simulink model "mysvm"  (R2017b)
settings: Solver=ode45  StartTime=0.0  StopTime=0.02  RelTol=1e-3  EnableMultiTasking=on
values from neighbouring files (symbols this model uses):
  N = svminput(5) - 1    [MLSVM_m_HD.m]    (also in PlotSpaceVector.m = block.DialogPrm(1).Data - 1)
undefined symbols (not defined in the file or in its folder): m
libraries: powerlib x9, powerlib_meascontrol x5, simulink x1
settings Model: Creator=吴鸿达  LastModifiedBy=AdamWu
settings DataIOCC: LimitDataPoints=on  SaveFormat=Array  ReturnWorkspaceOutputs=on
settings OptimizationCC: LifeSpan=inf
settings DebuggingCC: SolverPrmCheckMsg=warning  SFUnexpectedBacktrackingDiag=warning  SFNoUnconditionalDefaultTransitionDiag=warning  SFExecutionAtInitializationDiag=none
settings HardwareCC: ProdBitPerPointer=32  ProdBitPerSizeT=32  ProdBitPerPtrDiffT=32  ProdLargestAtomicFloat=None  ProdIntDivRoundTo=Undefined  ProdEndianess=Unspecified  ProdWordSize=32  ProdHWDeviceType=32-bit Generic
settings ModelReferenceCC: PropagateSignalLabelsOutOfModel=off
settings CodeAppCC: StateflowObjectComments=on
settings GRTTargetCC: TargetLangStandard=C89/C90 (ANSI)  GeneratePreprocessorConditionals=Disable all
settings ConfigComp: CovMetricSettings=dw  CovHtmlReporting=on  CovSaveCumulativeToWorkspaceVar=on  CovSaveSingleToWorkspaceVar=on  CovExternalEMLEnable=off  CovSFcnEnable=off
settings SimscapeCC: SimscapeNormalizeSystem=off

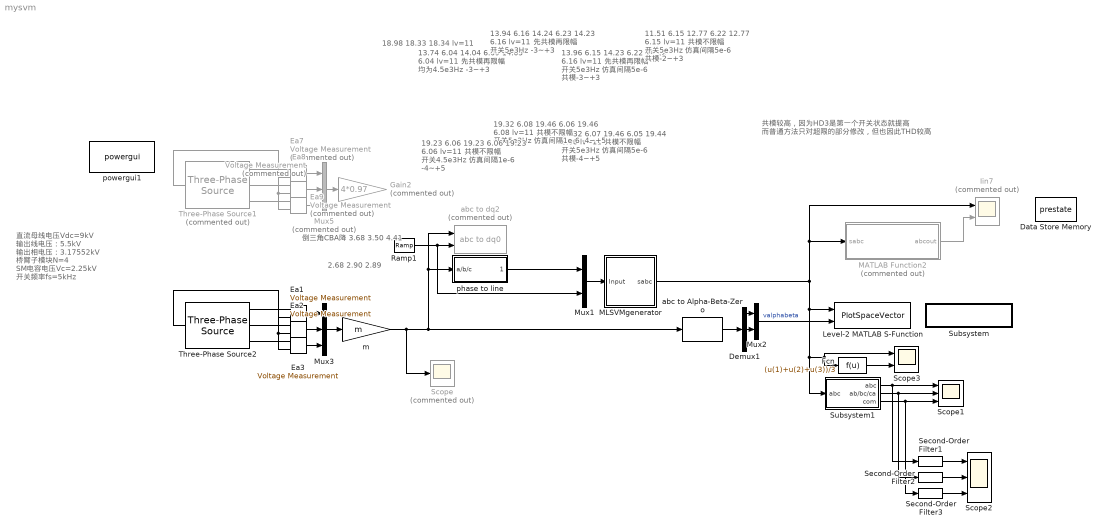
== system mysvm ==
  note: 18.98
      | 18.33
      | 18.34
      | lv=11
  note: 2.68 2.90 2.89
  note: 直流母线电压Vdc=9kV
      |
      | 输出线电压：5.5kV
      | 输出相电压：3.17552kV
      | 桥臂子模块N=4
      | SM电容电压Vc=2.25kV
      | 开关频率fs=5kHz
  note: 倒三角CBA降 3.68 3.50 4.41
  note: 13.74	6.04
      | 14.04	6.09
      | 14.05	6.04
      | lv=11
      | 先共模再限幅
      | 均为4.5e3Hz
      | -3~+3
  note: 13.94	6.16
      | 14.24	6.23
      | 14.23	6.16
      | lv=11
      | 先共模再限幅
      | 开关5e3Hz
      | -3~+3
  note: 13.96	6.15
      | 14.23	6.22
      | 14.22	6.16
      | lv=11
      | 先共模再限幅
      | 开关5e3Hz
      | 仿真间隔5e-6
      | 共模-3~+3
  note: 19.32	6.07
      | 19.46	6.05
      | 19.44	6.08
      | lv=11
      | 共模不限幅
      | 开关5e3Hz
      | 仿真间隔5e-6
      | 共模-4~+5
  note: 19.32	6.08
      | 19.46	6.06
      | 19.46	6.08
      | lv=11
      | 共模不限幅
      | 开关5e3Hz
      | 仿真间隔1e-6
      | -4~+5
  note: 19.23	6.06
      | 19.23	6.06
      | 19.23	6.06
      | lv=11
      | 共模不限幅
      | 开关4.5e3Hz
      | 仿真间隔1e-6
      | -4~+5
  note: 11.51	6.15
      | 12.77	6.22
      | 12.77	6.15
      | lv=11
      | 共模不限幅
      | 开关5e3Hz
      | 仿真间隔5e-6
      | 共模-2~+3
  note: 共模较高，因为HD3是第一个开关状态就提高
      | 而普通方法只对超限的部分修改，但也因此THD较高
  Data Store Memory : DataStoreMemory  DataStoreName=prestate  ReadBeforeWriteMsg=warning  WriteAfterWriteMsg=warning  WriteAfterReadMsg=warning  InitialValue=[0 0 0 0 0 0 0 1 0]  ShowAdditionalParam=off  OutDataTypeStr=double
  Demux1 : Demux  Outputs=3
  Ea1 : powerlib/Measurements/Voltage Measurement  PhasorSimulation=off  OutputType=Complex  PSBequivalent=0
  Ea2 : powerlib/Measurements/Voltage Measurement  PhasorSimulation=off  OutputType=Complex  PSBequivalent=0
  Ea3 : powerlib/Measurements/Voltage Measurement  PhasorSimulation=off  OutputType=Complex  PSBequivalent=0
  Ea7 : powerlib/Measurements/Voltage Measurement  Commented=on  PhasorSimulation=off  OutputType=Complex  PSBequivalent=0
  Ea8 : powerlib/Measurements/Voltage Measurement  Commented=on  PhasorSimulation=off  OutputType=Complex  PSBequivalent=0
  Ea9 : powerlib/Measurements/Voltage Measurement  Commented=on  PhasorSimulation=off  OutputType=Complex  PSBequivalent=0
  Fcn : Fcn  Expr=(u(1)+u(2)+u(3))/3
  Gain2 : Gain  Commented=on  Gain=4*0.97
  Iin7 : Scope  Commented=on  NumInputPorts=2
  Level-2 MATLAB S-Function : M-S-Function  FunctionName=PlotSpaceVector  Parameters=level, vdc, rate, normalized, plot, hexagon, sw, disabled  mask{disabled=off, level=N, rate=100, vdc=2/50, normalized=on, plot=1, hexagon=off, sw=off}
      mask prompts: disabled "Disable Plot"; level "Voltage Level"; rate "Plot Rate"; vdc "DC Link Voltage"; plot "Plot Number"; sw "Show Switching"
  MATLAB Function2 : MATLAB Function  Commented=on  TreatAsAtomicUnit=on
  MLSVMgenerator : Subsystem  mask{level=N, fs=1.5e3, vc=2.25e3, normalized=on, method=H-D3 Axis, dqorline=Line Voltages}
      mask prompts: level "Voltage Level"; fs "Switching Frequency"; vc "Capacitor Voltage"; method "Simplify Algorithm"; dqorline "Input Voltage Type"
      mask TypeOptions method: H-D Axis | g-h Axis | ab-bc-ca Axis | H-D3 Axis | D-Y (v2016) Axis | Rotated H-D Axis (Zero Common Voltage)
      mask TypeOptions dqorline: dq0 Voltages | Line Voltages | Phase Voltages
      mask DialogControl dqorline Tooltip: dq0 voltages means vd vq v0; line voltages means vab vbc vca
  Mux1 : Mux  Inputs=2
  Mux2 : Mux  Inputs=2
  Mux3 : Mux  Inputs=3
  Mux5 : Mux  Commented=on  Inputs=3
  Ramp1 : simulink/Sources/Ramp  slope=2*pi*50  start=0  X0=0
  Scope : Scope  Commented=on
  Scope1 : Scope  NumInputPorts=3
  Scope2 : Scope  NumInputPorts=3
  Scope3 : Scope  NumInputPorts=2
  Second-Order Filter1 : powerlib_meascontrol/Filters/Second-Order Filter  FilterType=Lowpass  Fo=1000  Zeta=0.707  Ts=0  Initialize=on  Vac_Init="[0,  0,  50]"  Vdc_Init=0  PlotResponse=off  FreqRange=[0, 2000, 1]
      settings: SourceProductName=Simscape Power Systems  SourceProductBaseCode=PS
  Second-Order Filter2 : powerlib_meascontrol/Filters/Second-Order Filter  FilterType=Lowpass  Fo=1000  Zeta=0.707  Ts=0  Initialize=on  Vac_Init="[0,  0,  50]"  Vdc_Init=0.5  PlotResponse=off  FreqRange=[0, 2000, 1]
      settings: SourceProductName=Simscape Power Systems  SourceProductBaseCode=PS
  Second-Order Filter3 : powerlib_meascontrol/Filters/Second-Order Filter  FilterType=Lowpass  Fo=1000  Zeta=0.707  Ts=0  Initialize=on  Vac_Init="[0,  0,  50]"  Vdc_Init=0.5  PlotResponse=off  FreqRange=[0, 2000, 1]
      settings: SourceProductName=Simscape Power Systems  SourceProductBaseCode=PS
  Subsystem : Subsystem  mask{filename=SVPWM_sFunction.m}
      settings: AttributesFormatString=\n  OpenFcn=open('F:\研究生\matlab\PlotSpaceVector.m')
      mask Display:
      | patch([0 1 1 0], [0 0 1 1],[0.2 0.6 0.9])
      | disp('plotspacevector.m')
  Subsystem1 : Subsystem  mask{N=N, normal=off}
      mask prompts: N "Voltage Level"; normal "Normalized"
  Three-Phase Source1 : powerlib/Electrical Sources/Three-Phase Source  Commented=on  InternalConnection=Yn  VoltagePhases=off  Voltage=1.59099e3  PhaseAngle=0  Voltage_phases=[25e3 25e3 25e3]/sqrt(3)  PhaseAngles_phases=[0 -120 +120]  Frequency=50  NonIdealSource=off  SpecifyImpedance=off  Resistance=0.8929  Inductance=1e-3  ShortCircuitLevel=100e6  BaseVoltage=25e3  XRratio=7  BusType=swing  Pref=10e3  Qref=0  Prefabc=[10e3, 10e3, 10e3]  Qrefabc=[0, 0, 0]  Qmin=-inf  Qmax=inf
  Three-Phase Source2 : powerlib/Electrical Sources/Three-Phase Source  InternalConnection=Yn  VoltagePhases=off  Voltage=sqrt(2)  PhaseAngle=0  Voltage_phases=[25e3 25e3 25e3]/sqrt(3)  PhaseAngles_phases=[0 -120 +120]  Frequency=50  NonIdealSource=off  SpecifyImpedance=off  Resistance=0.8929  Inductance=1e-3  ShortCircuitLevel=100e6  BaseVoltage=25e3  XRratio=7  BusType=swing  Pref=10e3  Qref=0  Prefabc=[10e3, 10e3, 10e3]  Qrefabc=[0, 0, 0]  Qmin=-inf  Qmax=inf
  abc to Alpha-Beta-Zero : powerlib_meascontrol/Transformations/abc to Alpha-Beta-Zero
      settings: SourceProductName=Simscape Power Systems
  abc to dq2 : powerlib_meascontrol/Transformations/abc to dq0  Commented=on  Alignment=90 degrees behind phase A axis
  m : Gain  Gain=m
  phase to line : Subsystem
  powergui1 : powerlib/powergui  Priority=1  SimulationMode=Discrete  SampleTime=0.5e-6  frequency=60  Iterations=50  frequencyindice=50  Pbase=100e6  ErrMax=1e-4  UnitsV=kV  UnitsW=MW  buscounter=0  FunctionMessages=off  echomessages=off  EnableUseOfTLC=off  CurrentSourceSwitches=off  DisableSnubberDevices=off  DisableRonSwitches=off  DisableVfSwitches=off  DisplayEquations=off  SolverType=Tustin/Backward Euler (TBE)  Interpol=off  ExternalGateDelay=off  methode=off  Ts=100  x0status=blocks  SPID=on  SwTol=0  HookPort=off  RestoreLinks=warning  ResistiveCurrentMeasurement=off  Frange=[0:2:500]  Ylog=off  Xlog=on  ShowGrid=off  save=off  variable=ZData  structure=SVMoutput  ZoomFFT=off  StartTime=0.00  cycles=1  DisplayStyle=1  fundamental=50  FreqAxis=on  MaxFrequency=15000  frequencyindicesteady=1  RmsSteady=1  display=off
  wires:
  Ramp1/1 -> Mux1/2, abc to dq2/2
  Ea9/1 -> Mux5/3
  Ea7/1 -> Mux5/1
  Ea8/1 -> Mux5/2
  Mux5/1 -> Gain2/1
  Mux1/1 -> MLSVMgenerator/1(Input)
  abc to Alpha-Beta-Zero/1 -> Demux1/1
  Demux1/1 -> Mux2/1
  Demux1/2 -> Mux2/2
  m/1 -> Scope/1, abc to dq2/1, phase to line/1(a/b/c), abc to Alpha-Beta-Zero/1
  Mux2/1 -> Level-2 MATLAB S-Function/2  "valphabeta"
  Subsystem1/2(ab/bc/ca) -> Scope1/2, Second-Order Filter2/1
  Subsystem1/3(com) -> Scope1/3, Second-Order Filter3/1
  Subsystem1/1(abc) -> Scope1/1, Second-Order Filter1/1
  MATLAB Function2/1(abcout) -> Iin7/2
  MLSVMgenerator/1(sabc) -> MATLAB Function2/1(sabc), Iin7/1, Fcn/1, Scope3/1, Subsystem1/1("abc "), Level-2 MATLAB S-Function/1
  Mux3/1 -> m/1
  Ea2/1 -> Mux3/2
  Ea1/1 -> Mux3/1
  Ea3/1 -> Mux3/3
  Second-Order Filter1/1 -> Scope2/1
  Second-Order Filter2/1 -> Scope2/2
  Second-Order Filter3/1 -> Scope2/3
  Fcn/1 -> Scope3/2
  phase to line/1(ab/bc/ca) -> Mux1/1
  connections:
  Ea9/LConn2 -- Three-Phase Source1/LConn1 -- Ea7/LConn2 -- Ea8/LConn2
  Three-Phase Source1/RConn1 -- Ea7/LConn1
  Three-Phase Source1/RConn2 -- Ea8/LConn1
  Three-Phase Source1/RConn3 -- Ea9/LConn1
  Ea3/LConn2 -- Ea2/LConn2 -- Ea1/LConn2 -- Three-Phase Source2/LConn1
  Three-Phase Source2/RConn2 -- Ea2/LConn1
  Three-Phase Source2/RConn3 -- Ea3/LConn1
  Three-Phase Source2/RConn1 -- Ea1/LConn1

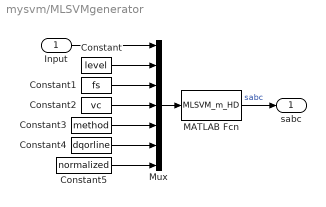
== system mysvm/MLSVMgenerator ==
  Input : Inport
  Constant : Constant  Value=level
  Constant1 : Constant  Value=fs
  Constant2 : Constant  Value=vc
  Constant3 : Constant  Value=method
  Constant4 : Constant  Value=dqorline
  Constant5 : Constant  Value=normalized
  MATLAB Fcn : MATLABFcn  MATLABFcn=MLSVM_m_HD  OutputSignalType=real
  Mux : Mux  Inputs=7
  sabc : Outport
  wires:
  MATLAB Fcn/1 -> sabc/1  "sabc"
  Input/1 -> Mux/1
  Constant1/1 -> Mux/3
  Constant/1 -> Mux/2
  Mux/1 -> MATLAB Fcn/1
  Constant2/1 -> Mux/4
  Constant3/1 -> Mux/5
  Constant4/1 -> Mux/6
  Constant5/1 -> Mux/7

== system mysvm/Subsystem ==

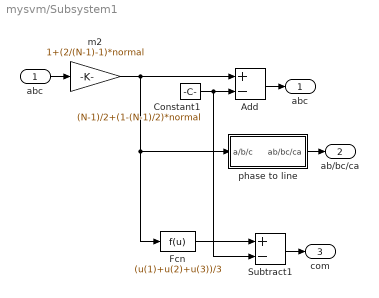
== system mysvm/Subsystem1 ==
  "abc " : Inport
  Add : Sum  Inputs=+-
  Constant1 : Constant  Value=(N-1)/2+(1-(N-1)/2)*normal
  Fcn : Fcn  Expr=(u(1)+u(2)+u(3))/3
  Subtract1 : Sum  Inputs=+-
  m2 : Gain  Gain=1+(2/(N-1)-1)*normal
  phase to line : Subsystem
  abc : Outport
  ab/bc/ca : Outport  Port=2
  com : Outport  Port=3
  wires:
  Subtract1/1 -> com/1
  "abc "/1 -> m2/1
  Fcn/1 -> Subtract1/1
  Constant1/1 -> Subtract1/2, Add/2
  m2/1 -> Add/1, phase to line/1(a/b/c), Fcn/1
  Add/1 -> abc/1
  phase to line/1(ab/bc/ca) -> ab/bc/ca/1

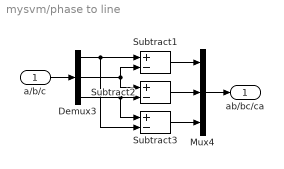
== system mysvm/phase to line ==
  a/b/c : Inport
  Demux3 : Demux  Outputs=3
  Mux4 : Mux  Inputs=3
  Subtract1 : Sum  Inputs=+-
  Subtract2 : Sum  Inputs=+-
  Subtract3 : Sum  Inputs=+-
  ab/bc/ca : Outport
  wires:
  Subtract2/1 -> Mux4/2
  Subtract1/1 -> Mux4/1
  Demux3/2 -> Subtract2/1, Subtract1/2
  a/b/c/1 -> Demux3/1
  Mux4/1 -> ab/bc/ca/1
  Demux3/3 -> Subtract2/2, Subtract3/1
  Subtract3/1 -> Mux4/3
  Demux3/1 -> Subtract1/1, Subtract3/2

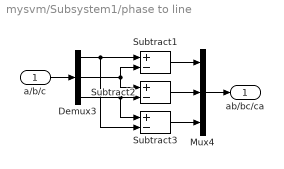
== system mysvm/Subsystem1/phase to line ==
  a/b/c : Inport
  Demux3 : Demux  Outputs=3
  Mux4 : Mux  Inputs=3
  Subtract1 : Sum  Inputs=+-
  Subtract2 : Sum  Inputs=+-
  Subtract3 : Sum  Inputs=+-
  ab/bc/ca : Outport
  wires:
  Subtract2/1 -> Mux4/2
  Subtract1/1 -> Mux4/1
  Demux3/2 -> Subtract2/1, Subtract1/2
  a/b/c/1 -> Demux3/1
  Mux4/1 -> ab/bc/ca/1
  Demux3/3 -> Subtract2/2, Subtract3/1
  Subtract3/1 -> Mux4/3
  Demux3/1 -> Subtract1/1, Subtract3/2

== matlab function mysvm/MATLAB Function2 ==
  settings: updateMethod=DISCRETE
  data: sabc input; abcout output; prestate data_store_memory
function abcout = TwoN_1(sabc)

sa = sabc(1);
sb = sabc(2);
sc = sabc(3);
N = 5;

global prestate
presa = prestate(1);
counta = prestate(2);
adc_ = prestate(3);
presb = prestate(4);
countb = prestate(5);
bdc_ = prestate(6);
presc = prestate(7);
countc = prestate(8);
cdc_ = prestate(9);

sa_ = sa - presa;
sb_ = sb - presb;
sc_ = sc - presc;
% nc = 0;

if sa_ == 0
    
else
    na = floor((sa + presa)/2);     % 0，1，2，。。。，N
    if mod(na, 2) == 0          % 偶数电平
        switch counta
            case 0
                adc_ = sa_;     % 直流电压同方向变化
            case 1
                adc_ = 0;       % 复原
            case 2
                adc_ = -sa_;    % 直流电压反方向变化
            case 3
                adc_ = 0;       % 复原
        end
    else                        % 奇数电平
        switch counta
            case 0
                adc_ = -sa_;
            case 1
                adc_ = 0;
            case 2
                adc_ = sa_;
            case 3
                adc_ = 0;
        end
    end
    
    counta = counta + 1;
    if counta > 3
        counta = 0;
    end
    
end

if sb_ == 0
    
else
    nb = floor((sb + presb)/2);
    if mod(nb, 2) == 0
        switch countb
            case 0
                bdc_ = sb_;
            case 1
                bdc_ = 0;
            case 2
                bdc_ = -sb_;
            case 3
                bdc_ = 0;
        end
    else
        switch countb
            case 0
                bdc_ = -sb_;
            case 1
                bdc_ = 0;
            case 2
                bdc_ = sb_;
            case 3
                bdc_ = 0;
        end
    end
    countb = countb + 1;
    if countb > 3
        countb = 0;
    end
end

if sc_ == 0
    
else
    nc = floor((sc + presc)/2);
    if mod(nc, 2) == 0
        switch countc
            case 0
                cdc_ = sc_;
            case 1
                cdc_ = 0;
            case 2
                cdc_ = -sc_;
            case 3
                cdc_ = 0;
        end
    else
        switch countc
            case 0
                cdc_ = -sc_;
            case 1
                cdc_ = 0;
            case 2
                cdc_ = sc_;
            case 3
                cdc_ = 0;
        end
    end
    countc = countc + 1;
    if countc > 3
        countc = 0;
    end
end

% if (sa_ ~= 0 || sb_ ~= 0 || sc_ ~= 0)
    prestate = [sa; counta; adc_; sb; countb; bdc_; sc; countc; cdc_];
% end
adc = N + adc_;         % 直流电压在N上下波动
bdc = N + bdc_;
cdc = N + cdc_;
sap = (adc - sa + N) / 2;
san = (adc + sa - N) / 2;
sbp = (bdc - sb + N) / 2;
sbn = (bdc + sb - N) / 2;
scp = (cdc - sc + N) / 2;
scn = (cdc + sc - N) / 2;
% abcout = [adc bdc cdc sap san sb_ bdc_ sc_ cdc_];
abcout = [adc bdc cdc sap san sbp sbn scp scn];

% global presabc;
% if any(presabc ~= sabc)
%     
% end
